simulink model "proje_p_2"  (R2016a)
settings: Solver=FixedStepAuto  StartTime=0.0  StopTime=10  FixedStep=STime  RelTol=1e-3
values from neighbouring files (symbols this model uses):
  STime = 1e-5    (= 1e-05)    [Part2_init.m]
libraries: powerlib x8, electricdrivelib x1, powerlib_meascontrol x1
settings Model: Creator=DELL  LastModifiedBy=gunge

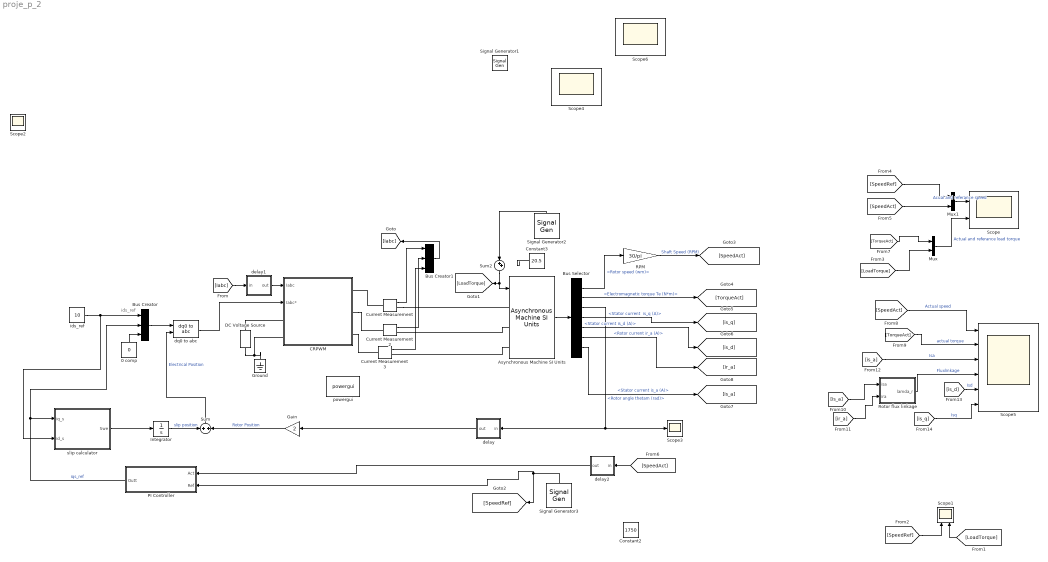
== system proje_p_2 ==
  note: ids_ref
  0 comp : Constant  Value=0
  Asynchronous Machine SI Units : powerlib/Machines/Asynchronous Machine SI Units  RotorType=Squirrel-cage  PresetModel=No  MechanicalLoad=Torque Tm  ShowDetailedParameters=on  ReferenceFrame=Stationary  Units=SI  MeasurementBus=off  NominalParameters=[3730 230 60]  Stator=[0.531 2.52e-3]  Rotor=[0.408 2.52e-3]  Cage1=[0.4155 0.002066]  Cage2=[0.4168 0.0003495]  Lm=84.7e-3  Mechanical=[1.1 0 2]  PolePairs=2  InitialConditions=[1 0 0 0 0 0 0 0]  SimulateSaturation=off  Saturation=[14.03593122, 27.81365428, 53.79336849, 72.68890987, 97.98006896, 148.6815601, 215.7428561, 302.9841135, 428.7778367 ; 230, 322, 414, 460, 506, 552, 598, 644, 690]  LoadFlowParameters=1492000  TsPowergui=0  TsBlock=-1  IterativeModel=Trapezoidal non iterative  IterativeDiscreteModel=Trapezoidal non iterative  Pmec=1.492e+006
  Bus Creator : BusCreator  Inputs=3
  Bus Creator1 : BusCreator  Inputs=3
  Bus Selector : BusSelector  OutputSignals="Mechanical.Rotor speed (wm),Mechanical.Electromagnetic torque Te (N*m),Mechanical.Rotor angle thetam (rad),Stator measurements.Stator current  is_q (A),Stator measurements.Stator current is_d (A),Rotor measurements.Rotor current ir_a (A),Stator measurements.Stator current is_a (A)"
  CRPWM : Subsystem
  Constant2 : Constant  Value=1750
  Constant3 : Constant  Value=20.5
  Current Measurement : powerlib/Measurements/Current Measurement  PhasorSimulation=off  OutputType=Complex  PSBequivalent=0
  Current Measurement2 : powerlib/Measurements/Current Measurement  PhasorSimulation=off  OutputType=Complex  PSBequivalent=0
  Current Measurement3 : powerlib/Measurements/Current Measurement  PhasorSimulation=off  OutputType=Complex  PSBequivalent=0
  DC Voltage Source : powerlib/Electrical Sources/DC Voltage Source  Amplitude=380  Measurements=None
  Gain : Gain  Gain=2
  Ground : powerlib/Elements/Ground  LConnTagsString=a
  Integrator : Integrator
  Mux : Mux  Inputs=2
  Mux1 : Mux  Inputs=2
  PI Controller : Subsystem
  RPM : Gain  Gain=30/pi
  Rotor flux linkage : MATLAB Function  TreatAsAtomicUnit=on
  Scope{,1,4,6} (4 alike) : Scope  NumInputPorts=2
  Scope3 : Scope
  Scope5 : Scope  NumInputPorts=6
  Signal Generator1 : SignalGenerator  WaveForm=square  Amplitude=-30.75  Frequency=0.1
  Signal Generator2 : SignalGenerator  WaveForm=square  Amplitude=-20  Frequency=0.1
  Signal Generator3 : SignalGenerator  WaveForm=square  Amplitude=-1740  Frequency=0.1
  Sum : Sum  Inputs=+|+
  Sum2 : Sum  Inputs=|++
  delay : Subsystem
  delay1 : Subsystem
  delay2 : Subsystem
  dq0 to abc : powerlib_meascontrol/Transformations/dq0 to abc  Alignment=90 degrees behind phase A axis
  ids_ref : Constant  Value=10
  powergui : powerlib/powergui  Priority=1  SimulationMode=Discrete  SolverType=Tustin/Backward Euler (TBE)  SampleTime=STime  frequency=60  SPID=off  DisableSnubberDevices=off  DisableRonSwitches=off  DisableVfSwitches=off  SwTol=0  DisplayEquations=off  Interpol=off  ExternalGateDelay=off  methode=off  Ts=10  FunctionMessages=off  echomessages=off  HookPort=off  EnableUseOfTLC=off  x0status=blocks  frequencyindice=60  Pbase=100e6  ErrMax=1e-4  Iterations=50  UnitsV=kV  UnitsW=MW  buscounter=0  RestoreLinks=warning  ResistiveCurrentMeasurement=off  Frange=[0:2:500]  Ylog=off  Xlog=on  ShowGrid=off  save=off  variable=ZData  structure=0  ZoomFFT=off  StartTime=0.0  cycles=1  DisplayStyle=1  fundamental=60  FreqAxis=off  MaxFrequency=1000  frequencyindicesteady=1  RmsSteady=1  display=off
  slip calculator : MATLAB Function  TreatAsAtomicUnit=on
  Scope2 : Scope
  wires:
  [Iabc] -> delay1/1(in)
  Asynchronous Machine SI Units/1 -> Bus Selector/1
  Bus Selector/3 -> delay/1(in), Scope3/1  "<Rotor angle thetam (rad)>"
  Gain/1 -> Sum/2  "Rotor Position"
  slip calculator/1(Swe) -> Integrator/1
  Integrator/1 -> Sum/1  "slip position"
  Bus Selector/1 -> RPM/1  "<Rotor speed (wm)>"
  Bus Selector/2 -> [TorqueAct]  "<Electromagnetic torque Te (N*m)>"
  ids_ref/1 -> Bus Creator/1, slip calculator/2(id_s)
  Bus Selector/4 -> [is_q]  "<Stator current  is_q (A)>"
  PI Controller/1(Outt) -> Bus Creator/2, slip calculator/1(iq_s)  "iqs_ref"
  Constant3/1 -> ?
  Sum2/1 -> [LoadTorque], Asynchronous Machine SI Units/1
  dq0 to abc/1 -> CRPWM/2("Iabc* ")
  Sum/1 -> dq0 to abc/2  "Electrical Position"
  Bus Creator1/1 -> [Iabc]
  delay2/1(out) -> PI Controller/1(Act)
  delay/1(out) -> Gain/1
  delay1/1(out) -> CRPWM/1(Iabc)
  [LoadTorque] -> Scope1/2
  Signal Generator3/1 -> PI Controller/2(Ref), [SpeedRef]
  [SpeedRef] -> Scope1/1
  [LoadTorque] -> Mux/2
  Mux/1 -> Scope/2  "Actual and referance load torque"
  Mux1/1 -> Scope/1  "Acual and referance speed"
  [SpeedRef] -> Mux1/1
  Bus Selector/6 -> [ir_a]  "<Rotor current ir_a (A)>"
  Bus Selector/7 -> [is_a]  "<Stator current is_a (A)>"
  0 comp/1 -> Bus Creator/3
  Bus Creator/1 -> dq0 to abc/1
  Current Measurement/1 -> Bus Creator1/1
  Current Measurement2/1 -> Bus Creator1/2
  Current Measurement3/1 -> Bus Creator1/3
  RPM/1 -> [SpeedAct]  "Shaft Speed (RPM)"
  [SpeedAct] -> Mux1/2
  [SpeedAct] -> delay2/1(in)
  [TorqueAct] -> Mux/1
  Rotor flux linkage/1(lamda_r) -> Scope5/4  "Fluxlinkage"
  [SpeedAct] -> Scope5/1  "Actual speed"
  [TorqueAct] -> Scope5/2  "actual torque"
  Bus Selector/5 -> [is_d]  "<Stator current is_d (A)>"
  [is_a] -> Rotor flux linkage/1(isa)
  [ir_a] -> Rotor flux linkage/2(ira)
  [is_a] -> Scope5/3  "Isa"
  [is_d] -> Scope5/5  "Isd"
  [is_q] -> Scope5/6  "Isq"
  Signal Generator2/1 -> Sum2/1
  connections:
  Ground/LConn1 -- CRPWM/LConn2 -- DC Voltage Source/LConn1
  DC Voltage Source/RConn1 -- CRPWM/LConn1
  Current Measurement/LConn1 -- CRPWM/RConn1
  Current Measurement/RConn1 -- Asynchronous Machine SI Units/LConn1
  Asynchronous Machine SI Units/LConn2 -- Current Measurement2/RConn1
  CRPWM/RConn2 -- Current Measurement2/LConn1
  Asynchronous Machine SI Units/LConn3 -- Current Measurement3/RConn1
  CRPWM/RConn3 -- Current Measurement3/LConn1

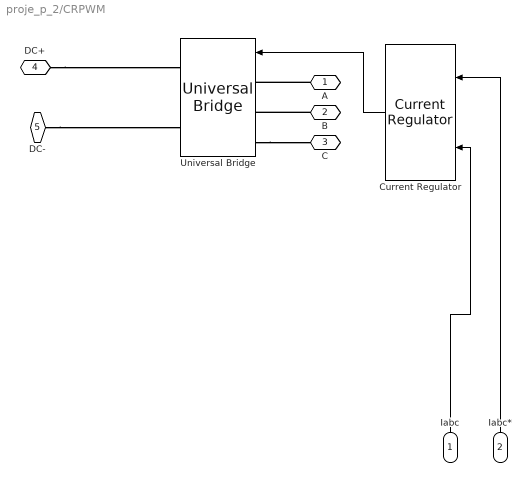
== system proje_p_2/CRPWM ==
  Iabc : Inport
  "Iabc* " : Inport  Port=2
  Current Regulator : electricdrivelib/Fundamental Drive Blocks/Vector Controller (PMSM)/Detailed_3ph/Current Regulator
  Universal Bridge : powerlib/Power Electronics/Universal Bridge  Arms=3  SnubberResistance=1e5  SnubberCapacitance=inf  Device=Ideal Switches  Ron=1e-3  Lon=0  ForwardVoltages="[  0.3  0.3  ]"  ForwardVoltage=0  GTOparameters=[ 10e-6 , 20e-6 ]  IGBTparameters=[ 1e-6 , 2e-6 ]  Measurements=None  Measurements_2=None  converterType=Rectifier
  A : PMIOPort  Port=1  Side=Right
  B : PMIOPort  Port=2  Side=Right
  C : PMIOPort  Port=3  Side=Right
  DC+ : PMIOPort  Port=4  Side=Left
  DC- : PMIOPort  Port=5  Side=Left
  wires:
  Current Regulator/1 -> Universal Bridge/1
  Iabc/1 -> Current Regulator/2
  "Iabc* "/1 -> Current Regulator/1
  connections:
  DC-/RConn1 -- Universal Bridge/RConn2
  A/RConn1 -- Universal Bridge/LConn1
  B/RConn1 -- Universal Bridge/LConn2
  Universal Bridge/LConn3 -- C/RConn1
  DC+/RConn1 -- Universal Bridge/RConn1

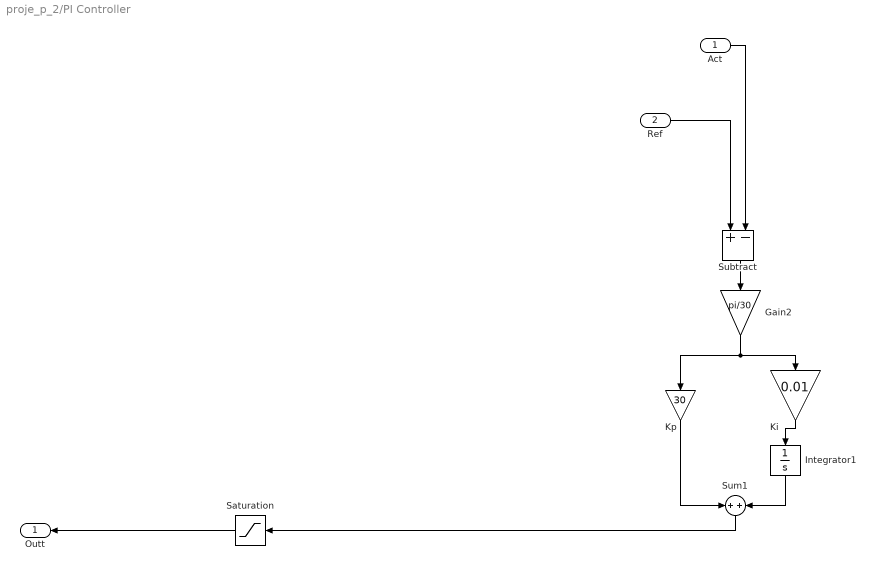
== system proje_p_2/PI Controller ==
  Act : Inport
  Ref : Inport  Port=2
  Gain2 : Gain  Gain=pi/30
  Integrator1 : Integrator
  Ki : Gain  Gain=0.01
  Kp : Gain  Gain=30
  Saturation : Saturate  UpperLimit=60  LowerLimit=-60
  Subtract : Sum  Inputs=+-
  Sum1 : Sum  Inputs=+|+
  Outt : Outport
  wires:
  Saturation/1 -> Outt/1
  Act/1 -> Subtract/2
  Subtract/1 -> Gain2/1
  Ki/1 -> Integrator1/1
  Kp/1 -> Sum1/1
  Gain2/1 -> Kp/1, Ki/1
  Sum1/1 -> Saturation/1
  Ref/1 -> Subtract/1
  Integrator1/1 -> Sum1/2

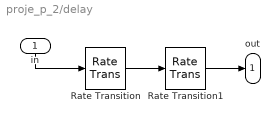
== system proje_p_2/delay ==
  in : Inport
  Rate Transition : RateTransition  OutPortSampleTime=150e-6
  Rate Transition1 : RateTransition
  out : Outport
  wires:
  in/1 -> Rate Transition/1
  Rate Transition/1 -> Rate Transition1/1
  Rate Transition1/1 -> out/1

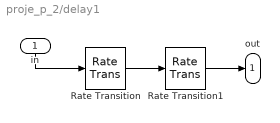
== system proje_p_2/delay1 ==
  in : Inport
  Rate Transition : RateTransition  OutPortSampleTime=150e-6
  Rate Transition1 : RateTransition
  out : Outport
  wires:
  in/1 -> Rate Transition/1
  Rate Transition/1 -> Rate Transition1/1
  Rate Transition1/1 -> out/1

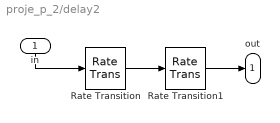
== system proje_p_2/delay2 ==
  in : Inport
  Rate Transition : RateTransition  OutPortSampleTime=150e-6
  Rate Transition1 : RateTransition
  out : Outport
  wires:
  in/1 -> Rate Transition/1
  Rate Transition/1 -> Rate Transition1/1
  Rate Transition1/1 -> out/1

== matlab function proje_p_2/slip calculator ==
  data: iq_s input; Swe output; id_s input
function Swe = fcn(iq_s,id_s)
%#codegen
Rr = 0.408;
Lr = (2.52+84.7)*1e-3;




Swe = Rr/Lr*iq_s/id_s;

== matlab function proje_p_2/Rotor flux linkage ==
  data: isa input; lamda_r output; ira input
function lamda_r = fcn(isa, ira)
%#codegen
Lm = 84.7e-3;
Lleak = 2.52e-3;

lamda_r = (isa+ira)*Lm + ira*Lleak;
